simulink model "alan2018"  (R2018b)
settings: Solver=FixedStepAuto  StartTime=0.0  StopTime=1  FixedStep=0.0001  RelTol=1e-3
values from neighbouring files (symbols this model uses):
  Cd = tf([(Kp + Kd * f) Kp * f], [1 f])    [alan.m]
  Gd = tf(c3, [1 c4 0])    [alan.m]
  Gss = ss(Dd * I)    [alan.m]
  I = tf([(v * dc) / (de * h)   v^2 / (de * h)], [1      0    -g / h])    [alan.m]
  K = place(A, B, polos)    [alan.m]
  L = place(Gss.A', Gss.C', polos)'    [alan.m]
libraries: simulink_extras x5
settings Model: Creator=lubuntu  LastModifiedBy=lubuntu

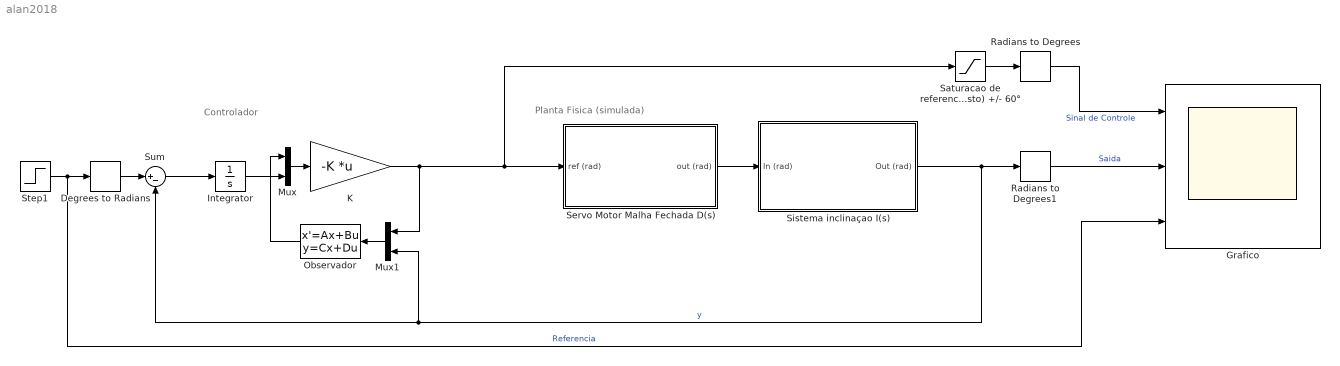
== system alan2018 ==
  note: Planta Fisica (simulada)
  note: Controlador
  Degrees to Radians : simulink_extras/Transformations/Degrees to Radians
  Grafico : Scope  NumInputPorts=3
  Integrator : Integrator
  K : Gain  Gain=-K  Multiplication=Matrix(K*u) (u vector)
  Mux : Mux  Inputs=2
  Mux1 : Mux  Inputs=2
  Observador : StateSpace  A=Gss.A-L*Gss.C  B=[Gss.B L]  C=eye(size(Gss.A, 1))  D=zeros(size(Gss.A,1), size(Gss.B,2)+1)  InitialCondition=0
  Radians to Degrees : simulink_extras/Transformations/Radians to Degrees
  Radians to Degrees1 : simulink_extras/Transformations/Radians to Degrees
  Saturacao de referencia do atuador (Limite Imposto) +/- 60° : Saturate  UpperLimit=60/180*pi  LowerLimit=-60/180*pi
  Servo Motor Malha Fechada D(s) : Subsystem
  Sistema inclinaçao I(s) : Subsystem
  Step1 : Step  Time=0.5  Before=8  After=0  SampleTime=0
  Sum : Sum  Inputs=|+-
  wires:
  Degrees to Radians/1 -> Sum/1
  Radians to Degrees/1 -> Grafico/1  "Sinal de Controle"
  Radians to Degrees1/1 -> Grafico/2  "Saida"
  Step1/1 -> Degrees to Radians/1, Grafico/3  "Referencia"
  Sistema inclinaçao I(s)/1(Out (rad)) -> Radians to Degrees1/1, Mux1/2, Sum/2  "y"
  Observador/1 -> Mux/1
  Sum/1 -> Integrator/1
  Mux/1 -> K/1
  Integrator/1 -> Mux/2
  Servo Motor Malha Fechada D(s)/1(out (rad)) -> Sistema inclinaçao I(s)/1(In (rad))
  Mux1/1 -> Observador/1
  K/1 -> Mux1/1, Servo Motor Malha Fechada D(s)/1(ref (rad)), Saturacao de referencia do atuador (Limite Imposto) +/- 60°/1
  Saturacao de referencia do atuador (Limite Imposto) +/- 60°/1 -> Radians to Degrees/1

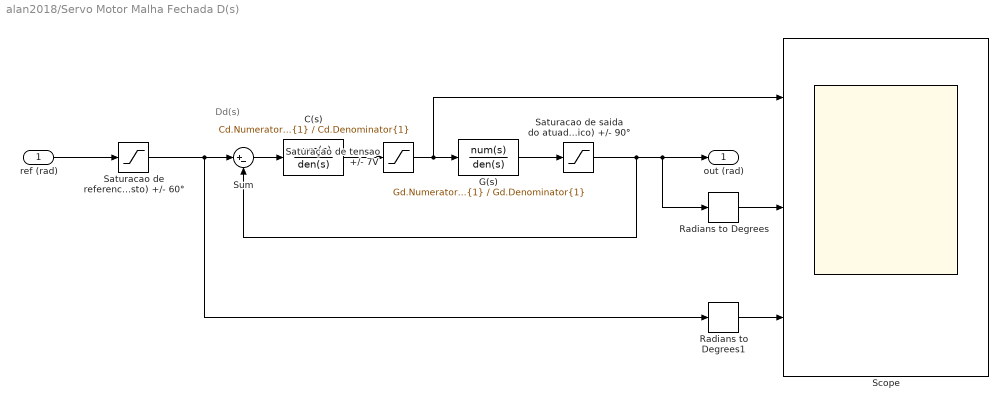
== system alan2018/Servo Motor Malha Fechada D(s) ==
  note: Dd(s)
  ref (rad) : Inport
  C(s) : TransferFcn  Numerator=Cd.Numerator{1}  Denominator=Cd.Denominator{1}
  G(s) : TransferFcn  Numerator=Gd.Numerator{1}  Denominator=Gd.Denominator{1}
  Radians to Degrees : simulink_extras/Transformations/Radians to Degrees
  Radians to Degrees1 : simulink_extras/Transformations/Radians to Degrees
  Saturacao de referencia do atuador (Limite Imposto) +/- 60° : Saturate  UpperLimit=60/180*pi  LowerLimit=-60/180*pi
  Saturacao de saida do atuador (limite fisico) +/- 90° : Saturate  UpperLimit=90/180*pi  LowerLimit=-90/180*pi
  Saturaçao de tensao +/- 7V : Saturate  UpperLimit=7  LowerLimit=-7
  Scope : Scope  NumInputPorts=3
  Sum : Sum  Inputs=|+-
  out (rad) : Outport
  wires:
  G(s)/1 -> Saturacao de saida do atuador (limite fisico) +/- 90°/1
  C(s)/1 -> Saturaçao de tensao +/- 7V/1
  Radians to Degrees/1 -> Scope/2
  Saturaçao de tensao +/- 7V/1 -> Scope/1, G(s)/1
  Sum/1 -> C(s)/1
  Radians to Degrees1/1 -> Scope/3
  ref (rad)/1 -> Saturacao de referencia do atuador (Limite Imposto) +/- 60°/1
  Saturacao de referencia do atuador (Limite Imposto) +/- 60°/1 -> Radians to Degrees1/1, Sum/1
  Saturacao de saida do atuador (limite fisico) +/- 90°/1 -> Sum/2, Radians to Degrees/1, out (rad)/1

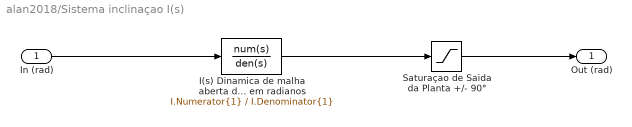
== system alan2018/Sistema inclinaçao I(s) ==
  In (rad) : Inport
  I(s) Dinamica de malha aberta do sistema de inclinacao Entrada e saida: Angulo em radianos : TransferFcn  Numerator=I.Numerator{1}  Denominator=I.Denominator{1}
  Saturaçao de Saida da Planta +/- 90° : Saturate  UpperLimit=90/180*pi  LowerLimit=-90/180*pi
  Out (rad) : Outport
  wires:
  Saturaçao de Saida da Planta +/- 90°/1 -> Out (rad)/1
  I(s) Dinamica de malha aberta do sistema de inclinacao Entrada e saida: Angulo em radianos/1 -> Saturaçao de Saida da Planta +/- 90°/1
  In (rad)/1 -> I(s) Dinamica de malha aberta do sistema de inclinacao Entrada e saida: Angulo em radianos/1
